simulink model "EE487_HW1_model"  (R2016a)
settings: Solver=VariableStepAuto  StartTime=0.0  StopTime=10.0  RelTol=1e-3
settings Model: Creator=Seth Barger  LastModifiedBy=Seth Barger

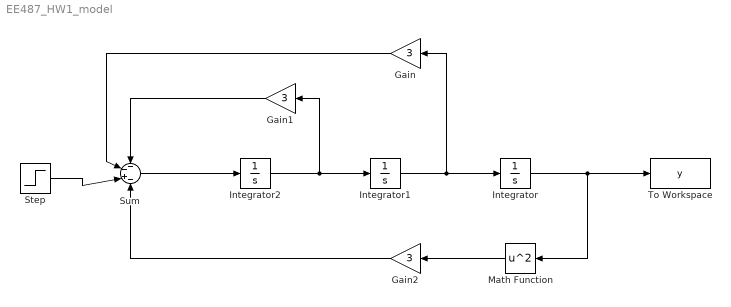
== system EE487_HW1_model ==
  Gain : Gain  Gain=3
  Gain1 : Gain  Gain=3
  Gain2 : Gain  Gain=3
  Integrator : Integrator
  Integrator1 : Integrator
  Integrator2 : Integrator
  Math Function : Math  Operator=square  SaturateOnIntegerOverflow=on
  Step : Step  SampleTime=0
  Sum : Sum  Inputs=--+-
  To Workspace : ToWorkspace  VariableName=y  SaveFormat=Timeseries  SampleTime=-1
  wires:
  Integrator/1 -> Math Function/1, To Workspace/1
  Integrator1/1 -> Gain/1, Integrator/1
  Integrator2/1 -> Gain1/1, Integrator1/1
  Sum/1 -> Integrator2/1
  Gain1/1 -> Sum/1
  Gain/1 -> Sum/2
  Math Function/1 -> Gain2/1
  Gain2/1 -> Sum/4
  Step/1 -> Sum/3
